simulink model "differ_equ"  (R2020b)
settings: Solver=VariableStepAuto  StartTime=0.0  StopTime=15  RelTol=1e-3
settings Model: Creator=99003736  LastModifiedBy=99003736

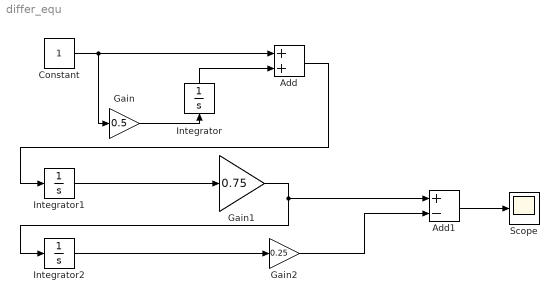
== system differ_equ ==
  Add : Sum
  Add1 : Sum  Inputs=+-
  Constant : Constant
  Gain : Gain  Gain=0.5
  Gain1 : Gain  Gain=0.75
  Gain2 : Gain  Gain=0.25
  Integrator : Integrator
  Integrator1 : Integrator
  Integrator2 : Integrator
  Scope : Scope
  wires:
  Gain/1 -> Integrator/1
  Constant/1 -> Add/1, Gain/1
  Integrator/1 -> Add/2
  Integrator1/1 -> Gain1/1
  Gain1/1 -> Add1/1, Integrator2/1
  Integrator2/1 -> Gain2/1
  Add/1 -> Integrator1/1
  Gain2/1 -> Add1/2
  Add1/1 -> Scope/1
